simulink subsystem "CONTROL"  (R2025b)
settings: Solver=VariableStepAuto  StartTime=0.0  StopTime=10.0  RelTol=1e-3
model mask{tacqAngThres=0, tacqKp=0, tacqKd=0, mtqMagneticGain=0, mtqResistance=0, mtqMaxVoltage=0, mtqMaxMagDip=0, mtqAllocationMatrix=0, magUpdateFreq=0}
  mask prompts: tacqAngThres "Angular error threshold [rad]"; tacqKp "Proportional gain (Kp)"; tacqKd "Derivative gain (Kd)"; mtqMagneticGain "Magnetic gain [Am2A-1]"; mtqResistance "Electrical resistance [Ohm]"; mtqMaxVoltage "Maximum voltage [V]"; mtqMaxMagDip "Maximum magnetic dipole [Am-2]"; mtqAllocationMatrix "Allocation Matrix"; magUpdateFreq "Update frequency [Hz]"
libraries: simulink x3
settings Model: Creator=antoniohernandez-rodiciomateos  LastModifiedBy=antoniohernandez-rodiciomateos

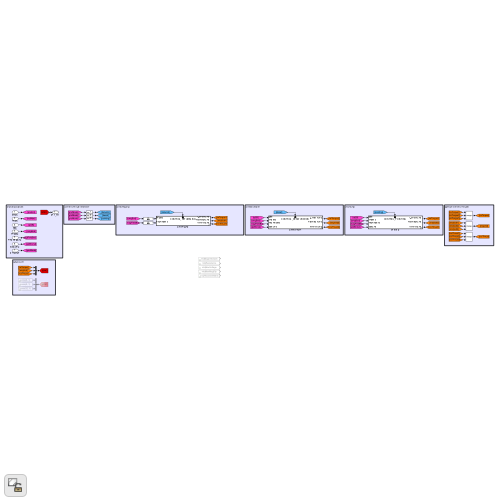
[thumbnail: Simulink's stored preview of the top-level diagram]
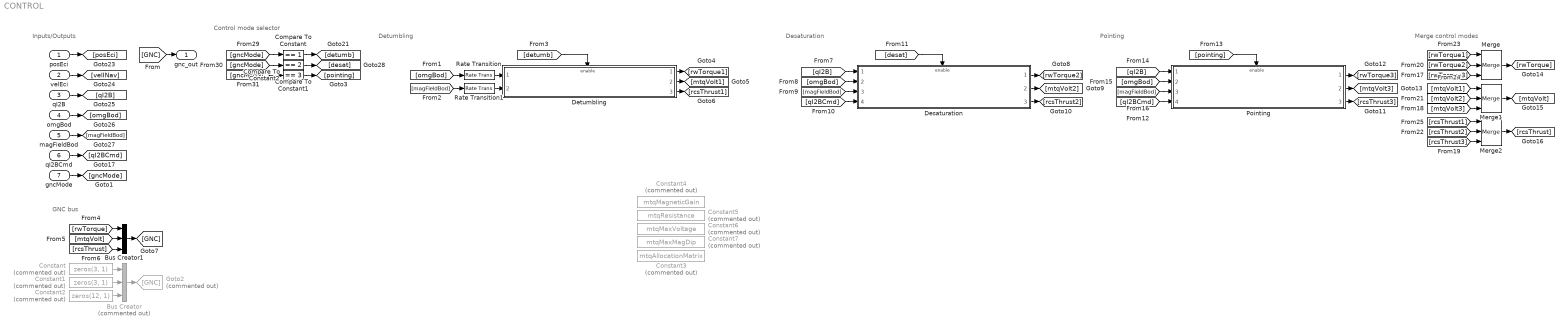
== system CONTROL ==
  note: Inputs/Outputs
  note: Control mode selector
  note: Detumbling
  note: Desaturation
  note: Pointing
  note: Merge control modes
  note: GNC bus
  posEci : Inport  OutDataTypeStr=double  PortDimensions=[3 1]
  velEci : Inport  Port=2  OutDataTypeStr=double  PortDimensions=[3 1]
  qI2B : Inport  Port=3  OutDataTypeStr=double  PortDimensions=[4 1]
  omgBod : Inport  Port=4  OutDataTypeStr=double  PortDimensions=[3 1]
  magFieldBod : Inport  Port=5  OutDataTypeStr=double  PortDimensions=[3 1]
  qI2BCmd : Inport  Port=6  OutDataTypeStr=double  PortDimensions=[4 1]
  gncMode : Inport  Port=7  OutDataTypeStr=double  PortDimensions=[1 1]
  Bus Creator : BusCreator  Commented=on  Inputs=3  OutDataTypeStr=Bus: gnc_bus  NonVirtualBus=on
      settings: InheritFromInputs=off
  Bus Creator1 : BusCreator  Inputs=3  OutDataTypeStr=Bus: gnc_bus  NonVirtualBus=on
      settings: InheritFromInputs=off
  Compare To Constant : simulink/Logic and Bit Operations/Compare To Constant  relop===  const=1  OutDataTypeStr=boolean
  Compare To Constant1 : simulink/Logic and Bit Operations/Compare To Constant  relop===  const=2  OutDataTypeStr=boolean
  Compare To Constant2 : simulink/Logic and Bit Operations/Compare To Constant  relop===  const=3  OutDataTypeStr=boolean
  Constant : Constant  Commented=on  Value=zeros(3, 1)
  Constant1 : Constant  Commented=on  Value=zeros(3, 1)
  Constant2 : Constant  Commented=on  Value=zeros(12, 1)
  Constant3 : Constant  Commented=on  Value=mtqAllocationMatrix
  Constant4 : Constant  Commented=on  Value=mtqMagneticGain
  Constant5 : Constant  Commented=on  Value=mtqResistance
  Constant6 : Constant  Commented=on  Value=mtqMaxVoltage
  Constant7 : Constant  Commented=on  Value=mtqMaxMagDip
  Desaturation : Subsystem  ReferencedSubsystem=CONTROL_DESATURATION
  Detumbling : Subsystem  ReferencedSubsystem=CONTROL_DETUMBLING
  Goto2 : Goto  Commented=on  GotoTag=GNC
  Merge : Merge  Inputs=3
  Merge1 : Merge  Inputs=3
  Merge2 : Merge  Inputs=3
  Pointing : Subsystem  ReferencedSubsystem=CONTROL_POINTING
  Rate Transition : RateTransition  OutPortSampleTime=1 / magUpdateFreq
  Rate Transition1 : RateTransition  OutPortSampleTime=1 / magUpdateFreq
  gnc_out : Outport  OutDataTypeStr=Bus: gnc_bus  PortDimensions=[1 1]
  wires:
  posEci/1 -> [posEci]
  qI2B/1 -> [qI2B]
  gncMode/1 -> [gncMode]
  velEci/1 -> [velINav]
  omgBod/1 -> [omgBod]
  qI2BCmd/1 -> [qI2BCmd]
  magFieldBod/1 -> [magFieldBod]
  [GNC] -> gnc_out/1
  [gncMode] -> Compare To Constant1/1
  [gncMode] -> Compare To Constant/1
  Compare To Constant/1 -> [detumb]
  Compare To Constant2/1 -> [pointing]
  Compare To Constant1/1 -> [desat]
  [gncMode] -> Compare To Constant2/1
  Detumbling/1 -> [rwTorque1]
  Detumbling/2 -> [mtqVolt1]
  Detumbling/3 -> [rcsThrust1]
  [detumb] -> Detumbling/Enable
  [rcsThrust] -> Bus Creator1/3
  [mtqVolt] -> Bus Creator1/2
  Constant2/1 -> Bus Creator/3
  [rwTorque] -> Bus Creator1/1
  Constant1/1 -> Bus Creator/2
  Bus Creator/1 -> Goto2/1
  Constant/1 -> Bus Creator/1
  Bus Creator1/1 -> [GNC]
  Rate Transition/1 -> Detumbling/1
  [omgBod] -> Rate Transition/1
  [magFieldBod] -> Rate Transition1/1
  Rate Transition1/1 -> Detumbling/2
  [magFieldBod] -> Pointing/3
  [desat] -> Desaturation/Enable
  [qI2B] -> Desaturation/1
  Merge2/1 -> [rcsThrust]
  [mtqVolt2] -> Merge1/2
  [qI2BCmd] -> Desaturation/4
  [mtqVolt3] -> Merge1/3
  Desaturation/3 -> [rcsThrust2]
  Pointing/3 -> [rcsThrust3]
  Merge/1 -> [rwTorque]
  [qI2BCmd] -> Pointing/4
  [rcsThrust1] -> Merge2/1
  [omgBod] -> Desaturation/2
  [magFieldBod] -> Desaturation/3
  Merge1/1 -> [mtqVolt]
  [omgBod] -> Pointing/2
  [rcsThrust3] -> Merge2/3
  [mtqVolt1] -> Merge1/1
  [rwTorque2] -> Merge/2
  Desaturation/2 -> [mtqVolt2]
  [qI2B] -> Pointing/1
  Pointing/1 -> [rwTorque3]
  Pointing/2 -> [mtqVolt3]
  [rwTorque1] -> Merge/1
  Desaturation/1 -> [rwTorque2]
  [rcsThrust2] -> Merge2/2
  [pointing] -> Pointing/Enable
  [rwTorque3] -> Merge/3
